simulink model "vardims_nestednonvirtualBus"  (Simulink 7.4)
settings: Solver=FixedStepDiscrete  StartTime=0.0  StopTime=10.0  FixedStep=0.2  RelTol=1e-3
PreLoadFcn:
  | load mvardims_bus2.mat;
CloseFcn:
  | clear a;
settings Model: Creator=djia  LastModifiedBy=jareta  ExtModeAutoUpdateStatusClock=off
settings DataIOCC: SaveFormat=StructureWithTime
settings OptimizationCC: InlineParams=on  CVOUCH=off  InitFltsAndDblsToZero=on  EfficientMapNaN2IntZero=off
settings DebuggingCC: StrictBusMsg=ErrorLevel1
settings SFSimCC: SimGenerateEmlReport=off
settings GRTTargetCC: TargetFcnLib=ansi_tfl_tmw.mat

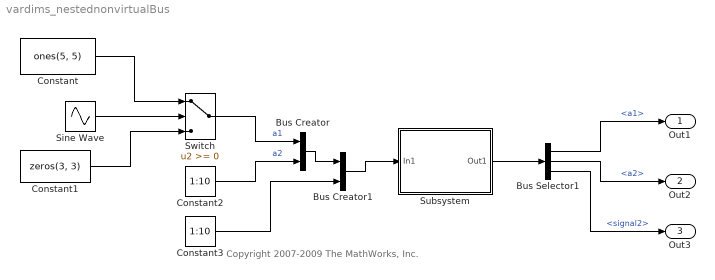
== system vardims_nestednonvirtualBus ==
  note: Copyright 2007-2009 The MathWorks, Inc.
  Bus Creator : BusCreator  Inputs=2  UseBusObject=on  NonVirtualBus=on
      settings: BusObject=a
  Bus Creator1 : BusCreator  Inputs=2  UseBusObject=on  NonVirtualBus=on
      settings: BusObject=b
  Bus Selector1 : BusSelector  OutputSignals=signal1.a1,signal1.a2,signal2
  Constant : Constant  Value=ones(5, 5)  OutDataType=sfix(16)  OutScaling=2^0
  Constant1 : Constant  Value=zeros(3, 3)  OutDataType=sfix(16)  OutScaling=2^0
  Constant2 : Constant  Value=1:10  OutDataType=sfix(16)  OutScaling=2^0  SampleTime=0.2
  Constant3 : Constant  Value=1:10  OutDataType=sfix(16)  OutScaling=2^0  SampleTime=0.2
  Sine Wave : Sin  Amplitude=1  Bias=0  Frequency=1  Phase=0  Samples=10  SampleTime=0.2  Offset=0
  Subsystem : Subsystem  TreatAsAtomicUnit=on
  Switch : Switch  OutDataType=sfix(16)  OutScaling=2^0  AllowDiffInputSizes=on
  Out1 : Outport  OutDataType=sfix(16)  OutScaling=2^0
  Out2 : Outport  Port=2  OutDataType=sfix(16)  OutScaling=2^0
  Out3 : Outport  Port=3  OutDataType=sfix(16)  OutScaling=2^0
  wires:
  Switch/1 -> Bus Creator/1  "a1"
  Constant/1 -> Switch/1
  Constant2/1 -> Bus Creator/2  "a2"
  Sine Wave/1 -> Switch/2
  Constant1/1 -> Switch/3
  Bus Creator/1 -> Bus Creator1/1
  Constant3/1 -> Bus Creator1/2
  Bus Creator1/1 -> Subsystem/1(In1)
  Subsystem/1(Out1) -> Bus Selector1/1
  Bus Selector1/1 -> Out1/1  "<a1>"
  Bus Selector1/2 -> Out2/1  "<a2>"
  Bus Selector1/3 -> Out3/1  "<signal2>"

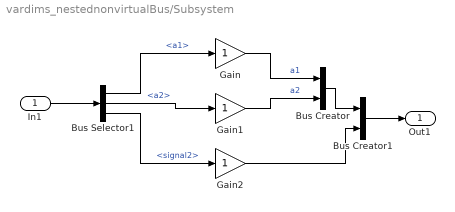
== system vardims_nestednonvirtualBus/Subsystem ==
  In1 : Inport
  Bus Creator : BusCreator  Inputs=2  UseBusObject=on
      settings: BusObject=a
  Bus Creator1 : BusCreator  Inputs=2  UseBusObject=on
      settings: BusObject=b
  Bus Selector1 : BusSelector  OutputSignals=signal1.a1,signal1.a2,signal2
  Gain : Gain  ParameterDataType=fixdt(1, 16)  ParameterScaling=2^0  OutDataType=fixdt(1, 16)  OutScaling=2^0
  Gain1 : Gain  ParameterDataType=fixdt(1, 16)  ParameterScaling=2^0  OutDataType=fixdt(1, 16)  OutScaling=2^0
  Gain2 : Gain  ParameterDataType=fixdt(1, 16)  ParameterScaling=2^0  OutDataType=fixdt(1, 16)  OutScaling=2^0
  Out1 : Outport
  wires:
  Bus Selector1/1 -> Gain/1  "<a1>"
  Bus Selector1/2 -> Gain1/1  "<a2>"
  Gain/1 -> Bus Creator/1  "a1"
  Gain1/1 -> Bus Creator/2  "a2"
  Bus Creator/1 -> Bus Creator1/1
  Gain2/1 -> Bus Creator1/2
  Bus Creator1/1 -> Out1/1
  In1/1 -> Bus Selector1/1
  Bus Selector1/3 -> Gain2/1  "<signal2>"
